simulink model "ADU_Integration_Y2016_simulation"  (R2016b)
settings: Solver=FixedStepDiscrete  StartTime=240  StopTime=300  FixedStep=0.01  RelTol=1e-3  EnableMultiTasking=on
PostLoadFcn:
  | , if any(exist('dsrtsu_mdlpostloadfcn', 'file') == [2, 3, 6]), try dsrtsu_mdlpostloadfcn('Execute', bdroot); catch fprintf('Error in PostLoadFcn (dsrtsu_mdlpostloadfcn) for model "%s":\n %s\n', bdroot, lasterr); end, end,
InitFcn:
  | load 'data/chi2_dat';
  | load 'data/innerLine_struct';
  | load 'data/middleLine_struct';
  | load 'data/outerLine_struct';
  | load 'data/innerLine';
  | load 'data/middleLine';
  | load 'data/outerLine';
  | load 'data/landmarks_patac_schimmel_ccw';
  | load 'data/patac_navi_array';
  | load 'data/sensor';
  | load 'data/map_struct';
  | addpath map_src
  | Integration_Parameter;
  | load 'TestData_001';
values from neighbouring files (symbols this model uses):
  TestData_001 =     [TestData_001.mat]
undefined symbols (not defined in the file or in its folder): a, chi2_dat, innerLine, landmarks_patac_schimmel_ccw, middleLine, outerLine, patac_navi_array, StartNum
libraries: simulink x36, rtican x1
(part 11 of 20)

== matlab function ADU_Integration_Y2016_simulation/Map/Map_Navigation ==
  data: global_landmarks output; vehicle_state output; object_list_update output; object_of_interest_id output; chi2_dat input; innerLine input; middleLine input; outerLine input; landmarks input; landmarks_in_proximity_id_in_front output [1..]; landmarks_in_proximity_id_in_rear output; odo_motion_v input; rtk_gps_lat input; rtk_gps_lon input; rtk_gps_yaw input; rtk_gps_ts input; sensor_data_raw input double size=[40 4]; object_list input double size=[127 26]; object_num input; chi2 data_store_memory; patac_navi input; maneuvers output; innerLaneMark output; middleLaneMark output; outerLaneMark output; ego_location output; odo_state_v output; t_in_utm output; x_in_utm output; y_in_utm output; a_in_utm output; delta_t output; x_last output; y_last output; v_last output; state_flag output; veh_ori_pos output; step_out output
%-------------------------------------------------------
% PATAC
% ADU
% SHD
% 
% Authors:  Binjian Xin
% Date   :  11-2016
%-------------------------------------------------------
% slam, explore data association algorithms
% hd_map: offline HD map orginal ground
% odo_motion: vehicle odometer data: odo_motion.x; odo_motion.y; odo_motion.yaw;
% sensor_data_raw: raw sensor data 40x4 [ID, x, y, MoveInfo]
% sensor_data_raw.srr[4] srr(1)-srr(4) are four SRR Radar raw data.
% srr(i).Measure --> [rho tita;...]
% srr(i).Rn --> [rho tita;...]c
% sensor_data_fusion: sensor fuison data; sensor_data_fusion
% 127x26
% [ID,RangeX,VelX,RangeY,VelY,MoveInfo,Width,Type,Fus_State,Confidence,
% P11,...P44]; FuseState Byte 9 for Lane Position Judge
% hd_map offline hd map, supposed to be converted to RTM 51r : wgs2utm(Lat,Lon,51,'N');
% hd_map.lanemarking1/lanemarking2/lanemarking3: three lanes, points in counterclockwise order; 1
% for left, 2 for middle, 3 for right;
% hd_map.landmark(:,5) (x,y,length, width, LandMarkType)
% rtk_gps: rtk_gps.[lat, lon, alt, yaw, pitch, roll, ts]
% 
%   enumeration
%   XCrossing_Stop (11) % 十字路口停止线
%   XCrossing_Start (12) % 十字路口目标车道进入线
%   TCrossing_Stop (21)%T字路口停止线
%   TCrossing_Start (22)%T字路口目标车道进入线
%   ZCrossing (30)%人行横道线
%   Stop_1 (51)%边线1（沿车道横向边线），摆渡车停车点。停车点可能没有实际的标记，请按估计的停车点选取位置，比如添加2号楼门口的停车点
%   Stop_2 (52)%边线2（沿车道横向边线）
%   LeftTurn_Stop (61)% 左转L形路口停止线
%   LeftTurn_Start (62)% 左转L形路口进入线
%   RightTurn_Stop (71)% 右转L形路口停止线
%   RightTurn_Start (72)% 右转L形路口进入线
%   ParkSlotOnRoad_Stop (81)% 路边停车位边线1（沿车道横向边线）
%   ParkSlotOnRoad_Start (82)% 路边停车位边线2（沿车道横向边线）
%   ParkSlotOffRoad (90)%  路外停车位，只需测量沿道路行驶方向的开始点和停止点
%   ParkSlotOffRoad_Start (91)%  路外停车位，只需测量沿道路行驶方向的开始点
%   ParkSlotOffRoad_Stop  (92)%  路外停车位，只需测量沿道路行驶方向的停止点
%   RoadChange (100)% 车道宽度变化点，如两点间距离暗示车道宽度，则此时两点选取应保证，两点连线同测量处的车道垂直，或者增加车道宽度的域。
%   SpeedLimit (110)%限速标志，点类型
%   GroundArrow (120)%地上箭头（参考EPM3的箭头位置定义），点类型
%   TrafficLight (130)%交通灯位置，点类型
%   UnClassified (180)%其他
%   end
%-------------------------------------------------------
%             t_in_utm,...
%             x_in_utm,...
%             y_in_utm,...
%             a_in_utm,...
%             delta_t,...
%             x_last,...
%             y_last,...
%             v_last,...
%             veh_ori_pos,...

function [global_landmarks,...
            vehicle_state, ...
            object_list_update, ...
            object_of_interest_id,...
            landmarks_in_proximity_id_in_front, ...
            landmarks_in_proximity_id_in_rear,...
            maneuvers, ...
            innerLaneMark,...
            middleLaneMark,...
            outerLaneMark,...
            ego_location, ...
            odo_state_v, ...
            t_in_utm,...
            x_in_utm,...
            y_in_utm,...
            a_in_utm,...
            delta_t,...
            x_last,...
            y_last,...
            v_last,...
            state_flag,...
            veh_ori_pos,...
            step_out] ...
    = slam_ekf_patac_map_pose_output...
        (chi2_dat, ...
        innerLine, ...
        middleLine, ...
        outerLine, ...
        landmarks,...
        odo_motion_v,...
        rtk_gps_lat, ...
        rtk_gps_lon, ...
        rtk_gps_yaw, ...
        rtk_gps_ts, ...
        sensor_data_raw, ...
        object_list, ...
        object_num, ...
        patac_navi)
global chi2;
persistent step veh_origin_pose configuration;
persistent x_in_utm_last y_in_utm_last a_in_utm_last t_in_utm_last a_rtk_offset;
persistent x_in_utm_last_meas y_in_utm_last_meas veh_vel_last wgs_ts_last;
% local_landmarks_ids = zeros(200,1);
persistent innerLine_lcs middleLine_lcs outerLine_lcs landmarks_lcs patac_navi_lcs object_list_lcs object_num_lcs object_list_update_lcs;
persistent landmarks_in_proximity_id_in_front_lcs landmarks_in_proximity_id_in_rear_lcs sensor_data_raw_lcs;
persistent object_of_interest_id_lcs ego_location_lcs;
%Convert rtk raw data to longitude, latitude, yaw in radian and ts in
%second
[wgs_lat,wgs_lon,wgs_yaw,wgs_ts_in_sec] = rtkraw2wgs (rtk_gps_lat, rtk_gps_lon, rtk_gps_yaw,rtk_gps_ts);
[x_in_utm,y_in_utm,~,~] = wgs2utm(wgs_lat,wgs_lon,51,'N');
wgs_yaw = 2*pi - wgs_yaw;


%rtk system --> VCS offset
x_rtk_offset = 0;

y_rtk_offset = 0;
a_rtk_offset = 90*pi/180;%rtk calibration info input!
x_in_utm = x_in_utm+x_rtk_offset;
y_in_utm = y_in_utm+y_rtk_offset;
a_in_utm = wgs_yaw + a_rtk_offset;
t_in_utm = wgs_ts_in_sec;

if a_in_utm>2*pi
    a_in_utm = a_in_utm-2*pi;
end

chi2 = chi2_dat;

persistent cnt;
if(isempty(cnt))
    cnt =0;
else
    cnt = cnt+1;
end

if (isempty(step) || cnt<100 )% first cycle
    step = 0;
    state_flag = 0;

    configuration = struct('ellipses',true,'tags',false,'odometry',true, ...
                            'noise',true,'alpha',0.99,'step_by_step',false,...
                            'people',false,'proximity',50, 'ground',1,'map',2,'observations',3,...
                            'compatibility',4,'ground_hypothesis',5,'hypothesis',6,...
                            'tables',7);
    configuration.step_by_step = true;   
    veh_origin_pose = struct('x_in_utm',0,'y_in_utm',0,'a_in_utm',0,'t_in_utm',0);   

    veh_origin_pose.x_in_utm = x_in_utm;% in Mercator
    veh_origin_pose.y_in_utm = y_in_utm;% in Mercator
    veh_origin_pose.a_in_utm = a_in_utm;
    veh_origin_pose.t_in_utm = t_in_utm;
    
    %Square One
    x_in_lcs = 0;
    y_in_lcs = 0;
    a_in_lcs = 0;
    t_in_lcs = 0;
    veh_pose = [0 0 0]';% x, y, yaw in LCS
    %standing still
    veh_vel = [0 0]';% V_x, V_y in LCS
    vehicle_state = [veh_pose; veh_vel];

    x_in_utm_last = x_in_utm;
    y_in_utm_last = y_in_utm;
    a_in_utm_last = a_in_utm;
    t_in_utm_last = t_in_utm;
    wgs_ts_last = wgs_ts_in_sec;
    x_in_utm_last_meas = x_in_utm;
    y_in_utm_last_meas = y_in_utm;
%     a_last = a_in_utm;
    veh_vel_last = [0 0]';

    innerLine_lcs = innerLine;
    middleLine_lcs = middleLine;
    outerLine_lcs = outerLine;
    landmarks_lcs = landmarks;
    patac_navi_lcs = patac_navi;
    object_list_lcs = object_list;
    object_num_lcs = object_num;
    object_list_update_lcs = object_list;
    landmarks_in_proximity_id_in_front_lcs = zeros(size(landmarks,1),1);
    landmarks_in_proximity_id_in_rear_lcs = zeros(size(landmarks,1),1); 
    object_of_interest_id_lcs = 0;
    sensor_data_raw_lcs = sensor_data_raw;
    ego_location_lcs = -1;
    
    landmarks_in_proximity_id_in_front = zeros(size(landmarks,1),1);
    landmarks_in_proximity_id_in_rear  = zeros(size(landmarks,1),1); 
    maneuvers = patac_navi;
    global_landmarks = landmarks;
    odo_state_v = odo_motion_v;
    step_out = 0;
    object_list_update = object_list;
    object_of_interest_id = 0;
    ego_location = -1; % due to invalid data from rtk ego locatoin cannot be determined.
    delta_t = 0;
    
    x_last = 0;
    y_last = 0;
    v_last = [0;0];
    veh_ori_pos = [veh_origin_pose.x_in_utm;veh_origin_pose.y_in_utm;veh_origin_pose.a_in_utm;veh_origin_pose.t_in_utm];
    
    innerLaneMark = innerLine.coordinate;
    middleLaneMark = middleLine.coordinate;
    outerLaneMark = outerLine.coordinate;    
    return;

end   
step = step +1;
if(step==1)
    innerLine_lcs = innerLine;
    middleLine_lcs = middleLine;
    outerLine_lcs = outerLine;
    innerLine_lcs.coordinate = innerLine.coordinate - ...
     [ones(size(innerLine.coordinate,1),1).*veh_origin_pose.x_in_utm,...
      ones(size(innerLine.coordinate,1),1).*veh_origin_pose.y_in_utm];
    middleLine_lcs.coordinate = middleLine.coordinate - ...
     [ones(size(middleLine.coordinate,1),1).*veh_origin_pose.x_in_utm,...
      ones(size(middleLine.coordinate,1),1).*veh_origin_pose.y_in_utm];
    outerLine_lcs.coordinate = outerLine.coordinate - ...
     [ones(size(outerLine.coordinate,1),1).*veh_origin_pose.x_in_utm,...
      ones(size(outerLine.coordinate,1),1).*veh_origin_pose.y_in_utm];

    %relocate landmarks in LCS, origin is the starting point.
    landmarks_lcs = landmarks;
    landmarks_lcs(:,1) = landmarks(:,1) - veh_origin_pose.x_in_utm;% landmarks in LCS!
    landmarks_lcs(:,2) = landmarks(:,2) - veh_origin_pose.y_in_utm;% landmarks in LCS!
    landmarks_lcs(:,3) = landmarks(:,3) - veh_origin_pose.x_in_utm;% landmarks in LCS!
    landmarks_lcs(:,4) = landmarks(:,4) - veh_origin_pose.y_in_utm;% landmarks in LCS!

    %relocate navigation maneuver list in LCS, origin is the starting point.
    patac_navi_lcs = patac_navi;
    patac_navi_lcs(:,1) = patac_navi(:,1) - veh_origin_pose.x_in_utm;%navigation maneuver in LCS!
    patac_navi_lcs(:,2) = patac_navi(:,2) - veh_origin_pose.y_in_utm;%navigation maneuver in LCS!

    veh_pose = [0 0 0]';% x, y, yaw in LCS
    %standing still
    veh_vel = [0 0]';% V_x, V_y in LCS
    vehicle_state = [veh_pose; veh_vel];    
    draw_map_nav_ground(innerLine_lcs.coordinate,innerLine_lcs.Vertex_index,...
                      middleLine_lcs.coordinate,middleLine_lcs.Vertex_index,...
                      outerLine_lcs.coordinate,outerLine_lcs.Vertex_index,...
                      landmarks_lcs, vehicle_state, patac_navi_lcs, configuration);

end

delta_t = (t_in_utm - t_in_utm_last);
if(abs(rtk_gps_lat)<1e-6 ...
   || abs(rtk_gps_lon)<1e-6 ...
   || abs(rtk_gps_ts)<1e-6...
   )%if invalid rtk data after initialization halfways due to rtk signal loss
    state_flag = 1; 
    t_in_lcs = (t_in_utm_last +0.01)-veh_origin_pose.t_in_utm;
    x_in_lcs = (x_in_utm_last+veh_vel_last(1)*0.01)-veh_origin_pose.x_in_utm;
    y_in_lcs = (y_in_utm_last+veh_vel_last(2)*0.01)-veh_origin_pose.y_in_utm;
    a_in_lcs = a_in_utm_last;
    veh_vel = veh_vel_last; 

    x_in_utm_last = x_in_utm_last + veh_vel_last(1)*0.01;
    y_in_utm_last = y_in_utm_last + veh_vel_last(2)*0.01;
    a_in_utm_last = a_in_utm;
    t_in_utm_last = t_in_utm_last+0.01;
%         veh_vel_last = veh_vel;
    wgs_ts_last = wgs_ts_in_sec;
%         x_in_utm_last_meas = x_in_utm;
%         y_in_utm_last_meas = y_in_utm;
else
    if(abs(wgs_ts_in_sec - wgs_ts_last)<1e-6)
        state_flag = 2;
        t_in_lcs = (t_in_utm_last +0.01)-veh_origin_pose.t_in_utm;
        x_in_lcs = (x_in_utm_last+veh_vel_last(1)*0.01)-veh_origin_pose.x_in_utm;
        y_in_lcs = (y_in_utm_last+veh_vel_last(2)*0.01)-veh_origin_pose.y_in_utm;
        a_in_lcs = a_in_utm_last;
        veh_vel = veh_vel_last; 

        x_in_utm_last = x_in_utm_last + veh_vel_last(1)*0.01;
        y_in_utm_last = y_in_utm_last + veh_vel_last(2)*0.01;
        a_in_utm_last = a_in_utm;
        t_in_utm_last = t_in_utm_last+0.01;
%             veh_vel_last = veh_vel;
        %wgs_ts_last = wgs_ts_in_sec;
    else
        state_flag = 3;
        t_in_lcs = t_in_utm - veh_origin_pose.t_in_utm;
        x_in_lcs = x_in_utm - veh_origin_pose.x_in_utm;
        y_in_lcs = y_in_utm - veh_origin_pose.y_in_utm;
        a_in_lcs = a_in_utm; %a_in_utm - veh_origin_pose.a_in_utm;
        %veh_vel = [(x_in_lcs-x_in_lcs_last)/0.01; (y_in_lcs-y_in_lcs_last)/0.01];%(ts_in_lcs - ts_in_lcs_last);
        veh_vel = [0;0];
        veh_vel(1) = (x_in_utm-x_in_utm_last_meas)*20;%(x_in_lcs-x_in_lcs_last)*100;
        veh_vel(2) = (y_in_utm-y_in_utm_last_meas)*20;%(y_in_lcs-y_in_lcs_last)*100;%(ts_in_lcs - ts_in_lcs_last);

        x_in_utm_last_meas = x_in_utm;
        y_in_utm_last_meas = y_in_utm;

        x_in_utm_last = x_in_utm;
        y_in_utm_last = y_in_utm;
        a_in_utm_last = a_in_utm;
        t_in_utm_last = t_in_utm;
        veh_vel_last = veh_vel;
        wgs_ts_last = wgs_ts_in_sec;
    end
end


x_last = x_in_utm_last;
y_last = y_in_utm_last;
v_last = veh_vel_last;
veh_ori_pos = [veh_origin_pose.x_in_utm;veh_origin_pose.y_in_utm;veh_origin_pose.a_in_utm;veh_origin_pose.t_in_utm];

veh_pose = [x_in_lcs y_in_lcs a_in_lcs]';% x, y, yaw in LCS
vehicle_state = [veh_pose; veh_vel];

%{
if isempty(step)
    step = 0;
    
    configuration = struct('ellipses',true,'tags',false,'odometry',true, ...
                            'noise',true,'alpha',0.99,'step_by_step',false,...
                            'people',false,'proximity',50, 'ground',1,'map',2,'observations',3,...
                            'compatibility',4,'ground_hypothesis',5,'hypothesis',6,...
                            'tables',7);
    configuration.step_by_step = true;                
    veh_origin_pose = struct('x_in_utm',0,'y_in_utm',0,'a_in_utm',0,'t_in_utm',0);   

    veh_origin_pose.x_in_utm = x_in_utm;% in Mercator
    veh_origin_pose.y_in_utm = y_in_utm;% in Mercator
    veh_origin_pose.a_in_utm = a_in_utm;
    veh_origin_pose.t_in_utm = t_in_utm;
    
    %Square One
    x_in_lcs = 0;
    y_in_lcs = 0;
    a_in_lcs = 0;
%   t_in_lcs = 0;
    veh_pose = [0 0 0]';% x, y, yaw in LCS
    %standing still
    veh_vel = [0 0]';% V_x, V_y in LCS
    vehicle_state = [veh_pose; veh_vel];
    
    x_in_utm_last = x_in_utm;
    y_in_utm_last = y_in_utm;
    a_in_utm_last = a_in_utm;
    t_in_utm_last = t_in_utm;
    veh_vel_last = [0 0]';
    wgs_ts_last = wgs_ts_in_sec;
    x_in_utm_last_meas = x_in_utm;
    y_in_utm_last_meas = y_in_utm;
    
    innerLine_lcs = innerLine;
    middleLine_lcs = middleLine;
    outerLine_lcs = outerLine;
    landmarks_lcs = landmarks;
    patac_navi_lcs = patac_navi;
    object_list_lcs = object_list;
    object_num_lcs = object_num;
    object_list_update_lcs = object_list;
    
    landmarks_in_proximity_id_in_front = zeros(size(landmarks,1),1);
    landmarks_in_proximity_id_in_rear  = zeros(size(landmarks,1),1); 
    landmarks_in_proximity_id_in_rear_lcs  = landmarks_in_proximity_id_in_front;
    landmarks_in_proximity_id_in_front_lcs = landmarks_in_proximity_id_in_rear;
    
    maneuvers = patac_navi_lcs;
    global_landmarks = landmarks;
    odo_state_v = odo_motion_v;
    object_list_update = object_list_update_lcs;
    object_of_interest_id = 0;
    ego_location = -1; % due to invalid data from rtk ego locatoin cannot be determined.
    return;    
end
%after first cycle  
if( step ==0 )%initialisation
    if(abs(rtk_gps_lat)<1e-6 ...
       || abs(rtk_gps_lon)<1e-6 ...
       || abs(rtk_gps_ts)<1e-6...
      )
        % invalid rtk after first cycle
        step = 0;
        veh_pose = [0 0 0]';% x, y, yaw in LCS
        %standing still
        veh_vel = [0 0]';% V_x, V_y in LCS
        vehicle_state = [veh_pose; veh_vel];

        landmarks_in_proximity_id_in_front = zeros(size(landmarks,1),1);
        landmarks_in_proximity_id_in_rear  = zeros(size(landmarks,1),1); 
        maneuvers = patac_navi_lcs;
        global_landmarks = landmarks;
        odo_state_v = odo_motion_v;
        object_list_update = object_list_update_lcs;
        object_of_interest_id = 0;
        ego_location = -1;% due to invalid data from rtk ego locatoin cannot be determined.
%             delta_t = 0;
%             x_last = x_in_utm_last;
%             y_last = y_in_utm_last;
%             v_last = veh_vel_last;
%             veh_ori_pos = [veh_origin_pose.x_in_utm;veh_origin_pose.y_in_utm;veh_origin_pose.a_in_utm;veh_origin_pose.t_in_utm];
        return;
    else% valid rtk after first cycle for initialization, initialization most probably in this branch
        step = 1;

        veh_origin_pose.x_in_utm = x_in_utm;% in Mercator
        veh_origin_pose.y_in_utm = y_in_utm;% in Mercator
        veh_origin_pose.a_in_utm = a_in_utm;
        veh_origin_pose.t_in_utm = t_in_utm;

        x_in_lcs = 0;
        y_in_lcs = 0;
        a_in_lcs = a_in_utm;
%           t_in_lcs = wgs_ts_in_sec - veh_origin_pose.t_in_utm;
        veh_vel =  [0 0]';%[x_in_lcs-x_in_lcs_last; y_in_lcs-y_in_lcs_last]/(ts_in_lcs - ts_in_lcs_last);
        veh_pose = [x_in_lcs y_in_lcs a_in_lcs]';% x, y, yaw in LCS
        vehicle_state = [veh_pose; veh_vel];
%             delta_t = 0;
%             x_last = x_in_utm_last;
%             y_last = y_in_utm_last;
%             v_last = veh_vel_last;
%             veh_ori_pos = [veh_origin_pose.x_in_utm;veh_origin_pose.y_in_utm;veh_origin_pose.a_in_utm;veh_origin_pose.t_in_utm];

        x_in_utm_last = x_in_utm;
        y_in_utm_last = y_in_utm;
        a_in_utm_last = a_in_utm;
        t_in_utm_last = t_in_utm;
        veh_vel_last = [0 0]';  
        wgs_ts_last = wgs_ts_in_sec;
        x_in_utm_last_meas = x_in_utm;
        y_in_utm_last_meas = y_in_utm;


        innerLine_lcs.coordinate = innerLine.coordinate - ...
         [ones(size(innerLine.coordinate,1),1).*veh_origin_pose.x_in_utm,...
          ones(size(innerLine.coordinate,1),1).*veh_origin_pose.y_in_utm];
        middleLine_lcs.coordinate = middleLine.coordinate - ...
         [ones(size(middleLine.coordinate,1),1).*veh_origin_pose.x_in_utm,...
          ones(size(middleLine.coordinate,1),1).*veh_origin_pose.y_in_utm];
        outerLine_lcs.coordinate = outerLine.coordinate - ...
         [ones(size(outerLine.coordinate,1),1).*veh_origin_pose.x_in_utm,...
          ones(size(outerLine.coordinate,1),1).*veh_origin_pose.y_in_utm];

        %relocate landmarks in LCS, origin is the starting point.
        landmarks_lcs(:,1) = landmarks(:,1) - veh_origin_pose.x_in_utm;% landmarks in LCS!
        landmarks_lcs(:,2) = landmarks(:,2) - veh_origin_pose.y_in_utm;% landmarks in LCS!
        landmarks_lcs(:,3) = landmarks(:,3) - veh_origin_pose.x_in_utm;% landmarks in LCS!
        landmarks_lcs(:,4) = landmarks(:,4) - veh_origin_pose.y_in_utm;% landmarks in LCS!

        %relocate navigation maneuver list in LCS, origin is the starting point.
        patac_navi_lcs(:,1) = patac_navi(:,1) - veh_origin_pose.x_in_utm;%navigation maneuver in LCS!
        patac_navi_lcs(:,2) = patac_navi(:,2) - veh_origin_pose.y_in_utm;%navigation maneuver in LCS!

        landmarks_in_proximity_id_in_front = zeros(size(landmarks,1),1);
        landmarks_in_proximity_id_in_rear  = zeros(size(landmarks,1),1); 
        object_list_update = object_list;
        object_of_interest_id = 0;
        ego_location = -1; % due to invalid data from rtk ego locatoin cannot be determined.

        maneuvers = patac_navi;
         global_landmarks = landmarks_lcs;
        odo_state_v = odo_motion_v;
        step_out = 0;
        return;         
    end
end% after initialization


if(abs(rtk_gps_lat)<1e-6 ...
   || abs(rtk_gps_lon)<1e-6 ...
   || abs(rtk_gps_ts)<1e-6...
   )%if invalid rtk data after initialization halfways due to rtk signal loss
%             t_in_lcs = (t_in_utm_last +0.01)-veh_origin_pose.t_in_utm;
    x_in_lcs = (x_in_utm_last+veh_vel_last(1)*0.01)-veh_origin_pose.x_in_utm;
    y_in_lcs = (y_in_utm_last+veh_vel_last(2)*0.01)-veh_origin_pose.y_in_utm;
    a_in_lcs = a_in_utm_last;
    veh_vel = veh_vel_last; 

    x_in_utm_last = x_in_utm_last+veh_vel_last(1)*0.01;
    y_in_utm_last = y_in_utm_last+veh_vel_last(2)*0.01;
%   a_in_utm_last = a_in_utm_last;
    t_in_utm_last = t_in_utm+0.01;
    veh_vel_last = veh_vel;
    wgs_ts_last = wgs_ts_in_sec;
%         x_in_utm_last_meas = x_in_utm;
%         y_in_utm_last_meas = y_in_utm;            
else
    if(abs(wgs_ts_in_sec - wgs_ts_last)<1e-6)
%         t_in_lcs = (t_in_utm_last +0.01)-veh_origin_pose.t_in_utm;
        x_in_lcs = (x_in_utm_last+veh_vel_last(1)*0.01)-veh_origin_pose.x_in_utm;
        y_in_lcs = (y_in_utm_last+veh_vel_last(2)*0.01)-veh_origin_pose.y_in_utm;
        a_in_lcs = a_in_utm_last;
        veh_vel = veh_vel_last; 
        x_in_utm_last = x_in_utm_last+veh_vel_last(1)*0.01;
        y_in_utm_last = y_in_utm_last+veh_vel_last(2)*0.01;
%               a_in_utm_last = a_in_utm_last;
        t_in_utm_last = t_in_utm+0.01;
%               veh_vel_last = veh_vel;
%               wgs_ts_last = wgs_ts_in_sec;
%               x_in_utm_last_meas = x_in_utm;
%               y_in_utm_last_meas = y_in_utm;
    else
%               t_in_lcs = t_in_utm - veh_origin_pose.t_in_utm;
        x_in_lcs = x_in_utm-veh_origin_pose.x_in_utm;
        y_in_lcs = y_in_utm-veh_origin_pose.y_in_utm;
        a_in_lcs = a_in_utm; %a_in_utm - veh_origin_pose.a_in_utm;
%                 veh_vel = [(x_in_utm-x_in_utm_last)/0.01; (y_in_utm-y_in_utm_last)/0.01];%(ts_in_lcs - ts_in_lcs_last);
        veh_vel = [(x_in_utm-x_in_utm_last); (y_in_utm-y_in_utm_last)]/(t_in_utm - t_in_utm_last);
%                 veh_vel = [0;0];
%                 veh_vel(1) = (x_in_utm-x_in_utm_last_meas)*20;%(x_in_lcs-x_in_lcs_last)*100;
%                 veh_vel(2) = (y_in_utm-y_in_utm_last_meas)*20;%(y_in_lcs-y_in_lcs_last)*100;%(ts_in_lcs - ts_in_lcs_last);

        x_in_utm_last_meas = x_in_utm;
        y_in_utm_last_meas = y_in_utm;

        x_in_utm_last = x_in_utm;
        y_in_utm_last = y_in_utm;
        a_in_utm_last = a_in_utm;
        t_in_utm_last = t_in_utm;
        veh_vel_last = veh_vel;
        wgs_ts_last = wgs_ts_in_sec;               
    end
end

%         delta_t = (t_in_utm - t_in_utm_last);
%         x_last = x_in_utm_last;
%         y_last = y_in_utm_last;
%         v_last = veh_vel_last;
%         veh_ori_pos = [veh_origin_pose.x_in_utm;veh_origin_pose.y_in_utm;veh_origin_pose.a_in_utm;veh_origin_pose.t_in_utm];

veh_pose = [x_in_lcs y_in_lcs a_in_lcs]';% x, y, yaw in LCS
vehicle_state = [veh_pose; veh_vel];
%}

if(mod(step,2)==1)
    %Relocate object list in LCS
    %SCS --> VCS offset 
    x_scs_offset = 5.24/2.0;%vehicle length 5.24m
    y_scs_offset = 0;%vehicle width 1.8m

    %VCS --> CCS (Control Coordinate System) offset 
    x_ccs_offset = 0;
    y_ccs_offset = 0;
    % x_offset = x_scs_offset+x_ccs_offset;
    % y_offset = y_scs_offset+y_ccs_offset;
	object_list_id = object_list(:,1);
	valid = find(object_list_id);
	object_num_meas = size(valid,1);

    object_list_lcs = object_list;
    object_num_lcs = object_num_meas;

    object_loc = [object_list(1:object_num_meas,2),object_list(1:object_num_meas,4)]';
    object_loc(1,:) = object_loc(1,:) + x_scs_offset;
    object_loc(2,:) = object_loc(2,:) + y_scs_offset;
    Tab = [ x_in_lcs; y_in_lcs; a_in_lcs];
    Pa = tpcomp(Tab, object_loc);
    object_list_lcs(1:object_num_meas,2)=Pa(1,:)';%object_list(:,2)+ x_scs_offset + x_in_lcs;%RangeX in LCS, displacement of VCS to SCS by 2.6m, half of vehicle length
    object_list_lcs(1:object_num_meas,4)=Pa(2,:)';%object_list(:,4)+ y_scs_offset + y_in_lcs;%RangeY in LCS

    object_vec = [object_list(1:object_num_meas,3),object_list(1:object_num_meas,5)]';
    Tab = [ veh_vel(1); veh_vel(2); a_in_lcs];
    Pb = tpcomp(Tab, object_vec);
    object_list_lcs(1:object_num_meas,3)=Pb(1,:)';%object_list(:,3)+ veh_vel(1);%VelX
    object_list_lcs(1:object_num_meas,5)=Pb(2,:)';%object_list(:,5)+ veh_vel(2);%VelY    

%    raw_loc = [sensor_data_raw(:,2),sensor_data_raw(:,3)]';
%    Tab = [ x_scs_offset + x_in_lcs; y_scs_offset + y_in_lcs; a_in_lcs];
%    Pa = tpcomp(Tab, raw_loc);
%    sensor_data_raw_lcs = sensor_data_raw;
%    sensor_data_raw_lcs(:,2)=Pa(1,:)';%object_list(:,2)+ x_scs_offset + x_in_lcs;%RangeX in LCS, displacement of VCS to SCS by 2.6m, half of vehicle length
%    sensor_data_raw_lcs(:,3)=Pa(2,:)';%object_list(:,4)+ y_scs_offset + y_in_lcs;%RangeY in LCS

    %find local landmarks
    option.firstTime=1;
    option.clockWise=0;  %0 for counter-clockwise，1 for clockwise    
    [landmarks_in_proximity_id_in_front_lcs, landmarks_in_proximity_id_in_rear_lcs] = quest_map4landmark (x_in_lcs, y_in_lcs, landmarks_lcs,middleLine_lcs.coordinate, middleLine_lcs.Vertex_index,configuration,option);

%     landmarks_in_proximity_id_in_front = landmarks_in_proximity_id_in_front_lcs;
%     landmarks_in_proximity_id_in_rear = landmarks_in_proximity_id_in_rear_lcs;
    %     sensor_data_raw(:,2)=sensor_data_raw(:,2)+ x0_offset + veh_origin_pose.x;%RangeX, displacement of VCS to SCS by 2.6m, half of vehicle length
    %     sensor_data_raw(:,3)=sensor_data_raw(:,3)+ y0_offset + veh_origin_pose.y;%RangeY

    %    [veh_pose, veh_vel] = slam_ekf_patac (inner, middle, outer, landmarks, ...
    %         odo_motion_x, odo_motion_y, odo_motion_yaw, ...

    %         rtk_gps_lat, rtk_gps_lon, rtk_gps_yaw, rtk_gps_ts, ...
    %         sensor_data_raw,...
    %         proximity);

    
end

if(mod(step,2)==0)
    %locate objects in lanes    
    %decide object list location in lanes
    option.firstTime=1;
    option.clockWise=0;  %0 for counter-clockwise，1 for clockwise
    object_list_update_lcs  = object_localization(object_list_lcs, object_num_lcs, innerLine_lcs.coordinate,innerLine_lcs.Vertex_index,...
                                                          middleLine_lcs.coordinate,middleLine_lcs.Vertex_index,...
                                                          outerLine_lcs.coordinate,outerLine_lcs.Vertex_index,...
                                                          option);
end

if(mod(step,2)==1)
    %find the closest object in ego lane (probably CIPV)
    option.firstTime=1;
    option.clockWise=0;  %0 for counter-clockwise，1 for clockwise    
    [obj_closest_in_path_ID, ~,ego_location_lcs] = objects_of_interest(object_list_update_lcs,object_num_lcs,...
            x_in_lcs, y_in_lcs, innerLine_lcs.coordinate, innerLine_lcs.Vertex_index,...
            middleLine_lcs.coordinate, middleLine_lcs.Vertex_index,...
            outerLine_lcs.coordinate, outerLine_lcs.Vertex_index, option);
    object_of_interest_id_lcs = obj_closest_in_path_ID;

    draw_observations_nav_ground(innerLine_lcs.coordinate, innerLine_lcs.Vertex_index,...
                                    middleLine_lcs.coordinate, middleLine_lcs.Vertex_index,...
                                    outerLine_lcs.coordinate, outerLine_lcs.Vertex_index,...
                                    landmarks_lcs, landmarks_in_proximity_id_in_front_lcs, ...
                                    landmarks_in_proximity_id_in_rear_lcs, vehicle_state, object_list_lcs, ...
                                    object_of_interest_id_lcs, sensor_data_raw_lcs, ...
                                    patac_navi_lcs,configuration);
end

maneuvers = patac_navi_lcs;
odo_state_v = odo_motion_v;
global_landmarks = landmarks_lcs;
landmarks_in_proximity_id_in_front = landmarks_in_proximity_id_in_front_lcs;
landmarks_in_proximity_id_in_rear = landmarks_in_proximity_id_in_rear_lcs;
object_list_update = object_list_update_lcs;
object_of_interest_id = object_of_interest_id_lcs;
ego_location = ego_location_lcs;
innerLaneMark = innerLine_lcs.coordinate;
middleLaneMark = middleLine_lcs.coordinate;
outerLaneMark = outerLine_lcs.coordinate;
step_out = step;

== matlab function ADU_Integration_Y2016_simulation/Path_Plan1/CordTransfer ==
  data: Info_MeGCd input; Info_MePGCd output size=1,6; RoadInfoPGCd output size=2,4; Info_FdGCd input; Info_FoGCd input; Info_LdGCd input; Info_LoGCd input; CurOpGCd input; LongDisLimitGCd input; RoadInfoGCd input; Info_FdPGCd output size=1,6; Info_FoPGCd output size=1,6; Info_LdPGCd output size=1,6; Info_LoPGCd output size=1,6; LongDisLimitPGCd output; CurOpPGCd output; PGCdInfo output size=1,3
function [Info_MePGCd,RoadInfoPGCd,Info_FdPGCd,Info_FoPGCd,Info_LdPGCd,Info_LoPGCd,LongDisLimitPGCd,CurOpPGCd,PGCdInfo] = CordTransfer(Info_MeGCd,Info_FdGCd,Info_FoGCd,Info_LdGCd,Info_LoGCd,CurOpGCd,LongDisLimitGCd,RoadInfoGCd)
%#codegen
%RoadInfo(1,1) = Info_Me(1);RoadInfo(1,2) = Info_Me(2);RoadInfo(1,3) = Info_Me(6);RoadInfo(1,4) = EgoLaneInfo(2);
    persistent CurOpTemp PGCXorig PGCYorig PGCThetaorig
    if isempty(CurOpTemp)
        CurOpTemp = 0;
    end
    if isempty(PGCXorig)
        PGCXorig = 0;
    end
    if isempty(PGCYorig)
        PGCYorig = 0;
    end
    if isempty(PGCThetaorig)
        PGCThetaorig = 0;
    end
    Info_MePGCd = [0 0 0 0 0 0];Info_FdPGCd = [0 0 0 0 0 0];Info_FoPGCd = [0 0 0 0 0 0];Info_LdPGCd = [0 0 0 0 0 0];Info_LoPGCd = [0 0 0 0 0 0];LongDisLimitPGCd = 0;RoadInfoPGCd = [0 0 0 0;0 0 0 0];PGCdInfo = [0 0 0];
    LongDisLimitPGCd = LongDisLimitGCd;CurOpPGCd = CurOpGCd;
    if abs(CurOpTemp - CurOpGCd) >1e-1
        CurOpTemp = CurOpGCd;
        PGCXorig = RoadInfoGCd(1,1);
        PGCYorig = RoadInfoGCd(1,2);
        PGCThetaorig = RoadInfoGCd(1,3);
    else
    end
    Info_MePGCd = Info_MeGCd;RoadInfoPGCd = RoadInfoGCd;Info_FdPGCd = Info_FdGCd;Info_FoPGCd = Info_FoGCd;Info_LdPGCd = Info_LdGCd;Info_LoPGCd = Info_LoGCd;
    % Transform only when there is an operation
    if CurOpGCd > 1e-1
    %     theta_rot = angle_in;
        %     x_outRot = (x_out - x_in)*cos(theta_rot) + (y_out - y_in)*sin(theta_rot);
        %     y_outRot = (y_out - y_in)*cos(theta_rot) - (x_out - x_in)*sin(theta_rot);    
        % X Y Rot and Move
        Info_MePGCd(1) = (Info_MeGCd(1) - PGCXorig)*cos(PGCThetaorig) + (Info_MeGCd(2) - PGCYorig)*sin(PGCThetaorig); 
        Info_MePGCd(2) = (Info_MeGCd(2) - PGCYorig)*cos(PGCThetaorig) - (Info_MeGCd(1) - PGCXorig)*sin(PGCThetaorig); 
        Info_FdPGCd(1) = (Info_FdGCd(1) - PGCXorig)*cos(PGCThetaorig) + (Info_FdGCd(2) - PGCYorig)*sin(PGCThetaorig); 
        Info_FdPGCd(2) = (Info_FdGCd(2) - PGCYorig)*cos(PGCThetaorig) - (Info_FdGCd(1) - PGCXorig)*sin(PGCThetaorig); 
        Info_FoPGCd(1) = (Info_FoGCd(1) - PGCXorig)*cos(PGCThetaorig) + (Info_FoGCd(2) - PGCYorig)*sin(PGCThetaorig); 
        Info_FoPGCd(2) = (Info_FoGCd(2) - PGCYorig)*cos(PGCThetaorig) - (Info_FoGCd(1) - PGCXorig)*sin(PGCThetaorig); 
        Info_LdPGCd(1) = (Info_LdGCd(1) - PGCXorig)*cos(PGCThetaorig) + (Info_LdGCd(2) - PGCYorig)*sin(PGCThetaorig); 
        Info_LdPGCd(2) = (Info_LdGCd(2) - PGCYorig)*cos(PGCThetaorig) - (Info_LdGCd(1) - PGCXorig)*sin(PGCThetaorig); 
        Info_LoPGCd(1) = (Info_LoGCd(1) - PGCXorig)*cos(PGCThetaorig) + (Info_LoGCd(2) - PGCYorig)*sin(PGCThetaorig); 
        Info_LoPGCd(2) = (Info_LoGCd(2) - PGCYorig)*cos(PGCThetaorig) - (Info_LoGCd(1) - PGCXorig)*sin(PGCThetaorig); 
        RoadInfoPGCd(1,1) = (RoadInfoGCd(1,1) - PGCXorig)*cos(PGCThetaorig) + (RoadInfoGCd(1,2) - PGCYorig)*sin(PGCThetaorig); 
        RoadInfoPGCd(1,2) = (RoadInfoGCd(1,2) - PGCYorig)*cos(PGCThetaorig) - (RoadInfoGCd(1,1) - PGCXorig)*sin(PGCThetaorig);    
        RoadInfoPGCd(2,1) = (RoadInfoGCd(2,1) - PGCXorig)*cos(PGCThetaorig) + (RoadInfoGCd(2,2) - PGCYorig)*sin(PGCThetaorig); 
        RoadInfoPGCd(2,2) = (RoadInfoGCd(2,2) - PGCYorig)*cos(PGCThetaorig) - (RoadInfoGCd(2,1) - PGCXorig)*sin(PGCThetaorig); 
        %Angle Rot
        Info_MePGCd(6) = Info_MeGCd(6) - PGCThetaorig;
        Info_FdPGCd(6) = Info_FdGCd(6) - PGCThetaorig;
        Info_FoPGCd(6) = Info_FoGCd(6) - PGCThetaorig;
        Info_LdPGCd(6) = Info_LdGCd(6) - PGCThetaorig;      
        Info_LoPGCd(6) = Info_LoGCd(6) - PGCThetaorig;
        RoadInfoPGCd(1,3) = RoadInfoGCd(1,3) - PGCThetaorig;
        RoadInfoPGCd(2,3) = RoadInfoGCd(2,3) - PGCThetaorig;
        PGCdInfo = [PGCXorig,PGCYorig,PGCThetaorig];   
    else
        PGCXorig = 0;
        PGCYorig = 0;
        PGCThetaorig = 0;        
    end
 
end

== matlab function ADU_Integration_Y2016_simulation/Path_Plan1/CordTransfer1 ==
  data: PGCdInfo input; VsPathPlan_h_positionPGC input; VsPathPlan_h_position output; VsPathPlan_h_MotionPGC input; TargetThetaLoPGC input; VsPathPlan_h_Motion output; TargetThetaLo output
function [VsPathPlan_h_position,VsPathPlan_h_Motion,TargetThetaLo] = CordTransfer(PGCdInfo,VsPathPlan_h_positionPGC,VsPathPlan_h_MotionPGC,TargetThetaLoPGC)
%#codegen
%RoadInfo(1,1) = Info_Me(1);RoadInfo(1,2) = Info_Me(2);RoadInfo(1,3) = Info_Me(6);RoadInfo(1,4) = EgoLaneInfo(2);
VsPathPlan_h_position = VsPathPlan_h_positionPGC;
VsPathPlan_h_Motion = VsPathPlan_h_MotionPGC;
TargetThetaLo = TargetThetaLoPGC;
end

== stateflow chart ADU_Integration_Y2016_simulation/Fusion_Model/Fusion_Block/Side_Fusion/RR_SRR_CoordinateAlig ==
  state [rangeX,rangeY] = TemporalAligRR(range,azimuth,W,L,InstallAngRRSRR) [function]
  (default) -> (junction 95) : {
      | k=0;
      | RRSRR_Output=0;
      | }
  (junction 95) -> (junction 98) [order 1] : [k<10]
  (junction 98) -> (junction 104) [order 1] : [RRSRR_Input[k][0]!=0]
  (junction 101) -> (junction 95) : {
      | k++;
      | }
  (junction 95) -> (junction 96) [order 2] : {
      | SideFusion;
      | }
  (junction 98) -> (junction 101) [order 2]
  (junction 104) -> (junction 106) : {
      | RRSRR_Output[k][0]=RRSRR_Input[k][0];%Target ID
      | [RRSRR_Output[k][1],RRSRR_Output[k][2]]=TemporalAligRR(RRSRR_Input[k][1],RRSRR_Input[k][2],W,L,InstallAng*3.1415/180);
      | RRSRR_Output[k][3]=RRSRR_Input[k][4]; %Target DynamicMode
      | }
  (junction 106) -> (junction 101)
  data: range function_input; rangeX function_output; rangeY function_output; azimuth function_input; W function_input double size=1; L function_input double size=1; InstallAngRRSRR function_input double size=1; RRSRR_Input input double size=[10 5]; RRSRR_Output output double size=[10 4]; k local double size=1 =0; L constant double =5.2; W constant double =1.8; InstallAng constant double =60
  events: SRR_Trig input EITHER_EDGE_EVENT; SideFusion output FUNCTION_CALL_EVENT

== stateflow chart ADU_Integration_Y2016_simulation/LogData/Sensor_ESR/Chart ==
  (default) -> (junction 14) : {
      | k=0;
      | TargetNum=0;
      | DataOutput=0;
      | }
  (junction 14) -> (junction 25) [order 1] : [k<64]
  (junction 25) -> (junction 30) [order 1] : [DataInput[k][3]!=0]
  (junction 28) -> (junction 14) : {
      | k++;
      | }
  (junction 14) -> (junction 16) [order 2]
  (junction 25) -> (junction 28) [order 2]
  (junction 30) -> (junction 33) : {
      | DataOutput[TargetNum][0]=DataInput[k][0];
      | DataOutput[TargetNum][1]=DataInput[k][1];
      | DataOutput[TargetNum][2]=DataInput[k][2];
      | DataOutput[TargetNum][3]=DataInput[k][3];
      | TargetNum++;
      | }
  (junction 33) -> (junction 28)
  (junction 16) -> (junction 17)
  data: DataInput input size=[64 4]; DataOutput output double size=[64 4]; k local double size=1 =0; TargetNum local double size=1 =0
  events: Trigger input EITHER_EDGE_EVENT

== stateflow chart ADU_Integration_Y2016_simulation/LogData/LF_SRR_Data/Chart ==
  (default) -> (junction 13)
  (junction 13) -> (junction 14) [order 1] : [Trig != preTrig]
  (junction 13) -> (junction 15) [order 2]
  (junction 14) -> (junction 16) : {
      | DataOutput=DataInput;
      | Time_out=Time;
      | }
  (junction 16) -> (junction 15)
  (junction 15) -> (junction 17) : {
      | preTrig=Trig;
      | }
  data: Trig input; DataInput input size=[10 5]; DataOutput output double size=[10 5]; Time input; preTrig local double; Time_out output double

== stateflow chart ADU_Integration_Y2016_simulation/LogData/Sensor_ESR/Chart2 ==
  state B
  state B1
  (default) -> B : {count=0;}
  B -> B1 : {
      | count=count+1;
      | }
  B1 -> B : {
      | count=count-1;
      | }
  data: count output double
  events: event input FUNCTION_CALL_EVENT

== stateflow chart ADU_Integration_Y2016_simulation/Fusion_Model/Fusion_Block/Side_Fusion/SRR_Data_Out ==
  (default) -> (junction 113) : {
      | k=0;
      | SRR_Data=0;
      | SideFusNum=0;
      | }
  (junction 113) -> (junction 115) [order 1] : [k<10]
  (junction 118) -> (junction 113) : {
      | k++;
      | }
  (junction 113) -> (junction 129) [order 2] : {
      | k=0;
      | }
  (junction 115) -> (junction 118) : {
      | SRR_Data[SideFusNum][0]=LFSRR_Input[k][0];SRR_Data[SideFusNum][1]=LFSRR_Input[k][1];
      | SRR_Data[SideFusNum][2]=LFSRR_Input[k][2];SRR_Data[SideFusNum][3]=LFSRR_Input[k][3];
      | SideFusNum=SideFusNum+1;
      | }
  (junction 129) -> (junction 136) [order 1] : [k<10]
  (junction 140) -> (junction 129) : {
      | k++;
      | }
  (junction 129) -> (junction 151) [order 2] : {
      | k=0;
      | }
  (junction 136) -> (junction 140) : {
      | SRR_Data[SideFusNum][0]=RFSRR_Input[k][0];SRR_Data[SideFusNum][1]=RFSRR_Input[k][1];
      | SRR_Data[SideFusNum][2]=RFSRR_Input[k][2];SRR_Data[SideFusNum][3]=RFSRR_Input[k][3];
      | SideFusNum=SideFusNum+1;
      | }
  (junction 151) -> (junction 149) [order 1] : [k<10]
  (junction 145) -> (junction 151) : {
      | k++;
      | }
  (junction 151) -> (junction 160) [order 2] : {
      | k=0;
      | }
  (junction 149) -> (junction 145) : {
      | SRR_Data[SideFusNum][0]=LRSRR_Input[k][0];SRR_Data[SideFusNum][1]=LRSRR_Input[k][1];
      | SRR_Data[SideFusNum][2]=LRSRR_Input[k][2];SRR_Data[SideFusNum][3]=LRSRR_Input[k][3];
      | SideFusNum=SideFusNum+1;
      | }
  (junction 160) -> (junction 164) [order 1] : [k<10]
  (junction 159) -> (junction 160) : {
      | k++;
      | }
  (junction 160) -> (junction 172) [order 2]
  (junction 164) -> (junction 159) : {
      | SRR_Data[SideFusNum][0]=RRSRR_Input[k][0];SRR_Data[SideFusNum][1]=RRSRR_Input[k][1];
      | SRR_Data[SideFusNum][2]=RRSRR_Input[k][2];SRR_Data[SideFusNum][3]=RRSRR_Input[k][3];
      | SideFusNum=SideFusNum+1;
      | }
  data: LFSRR_Input input double size=[10 4]; RFSRR_Input input double size=[10 4]; LRSRR_Input input double size=[10 4]; RRSRR_Input input double size=[10 4]; SRR_Data output double size=[40 4]; k local double size=1 =0; count local double size=1 =0; SideFusNum local double size=1 =0

== matlab function ADU_Integration_Y2016_simulation/Path_Plan1/InterSectionPathPlanningModule/MATLAB Function ==
  data: CurOp input; TrigFlg output
function TrigFlg = OpTrigJudge(CurOp)
%#codegen
    %Operation 0 NA    %Operation 1 RT    %Operation 2 LT    %Operation 3 ST    %Operation 4 PK    %Operation 5 LC    %Operation 6 Transition
    persistent TrigEventEdge
    if isempty(TrigEventEdge)
        TrigEventEdge = 0;
    end
    TrigFlg = 0;
    if (abs(CurOp - 1)<1e-1) || ( abs(CurOp - 2)<1e-1)  
        TrigEdgeResCur = 1;
    else
        TrigEdgeResCur = 0;  
    end

    if ((abs(TrigEventEdge - TrigEdgeResCur) > 1e-1)) 
        if (TrigEdgeResCur > 1e-1)
            TrigFlg = 1;
        else
        end
        TrigEventEdge = TrigEdgeResCur;
    else
        TrigFlg = 0;
    end 
end

== stateflow chart ADU_Integration_Y2016_simulation/LogData/RF_SRR_Data/Chart ==
  (default) -> (junction 13)
  (junction 13) -> (junction 14) [order 1] : [Trig != preTrig]
  (junction 13) -> (junction 15) [order 2]
  (junction 14) -> (junction 16) : {
      | DataOutput=DataInput;
      | Time_out=Time;
      | }
  (junction 16) -> (junction 15)
  (junction 15) -> (junction 17) : {
      | preTrig=Trig;
      | }
  data: Trig input; DataInput input size=[10 5]; DataOutput output double size=[10 5]; Time input; preTrig local double; Time_out output double

== matlab function ADU_Integration_Y2016_simulation/Path_Plan1/InterSectionPathPlanningModule/MATLAB Function1 ==
  data: RoadInfo input; x_in output; y_in output; angle_in output; x_out output; y_out output; angle_out output; W_in output; W_out output
function [x_in,y_in,angle_in,x_out,y_out,angle_out,W_in,W_out] = RoadInfoDistribute(RoadInfo)
%#codegen
%         RoadInfo(1,1) = Info_Me(1);RoadInfo(1,2) = Info_Me(2);RoadInfo(1,3) = Info_Me(6);RoadInfo(1,4) = EgoLaneInfo(2);
%         RoadInfo(2,:) = [EgoLaneInfo(3),EgoLaneInfo(4),EgoLaneInfo(1),EgoLaneInfo(2)]; 
    x_in = RoadInfo(1,1);y_in = RoadInfo(1,2);angle_in = RoadInfo(1,3);W_in = RoadInfo(1,4);
    x_out = RoadInfo(2,1);y_out = RoadInfo(2,2);angle_out = RoadInfo(2,3); W_out = RoadInfo(2,4);
end

== stateflow chart ADU_Integration_Y2016_simulation/LogData/LR_SRR_Data/Chart ==
  (default) -> (junction 13)
  (junction 13) -> (junction 14) [order 1] : [Trig != preTrig]
  (junction 13) -> (junction 15) [order 2]
  (junction 14) -> (junction 16) : {
      | DataOutput=DataInput;
      | Time_out=Time;
      | }
  (junction 16) -> (junction 15)
  (junction 15) -> (junction 17) : {
      | preTrig=Trig;
      | }
  data: Trig input; DataInput input size=[10 5]; DataOutput output double size=[10 5]; Time input; preTrig local double; Time_out output double
